simulink model "simple"  (R2016a)
settings: Solver=VariableStepAuto  StartTime=0.0  StopTime=100  FixedStep=0.01  MaxStep=0.01  RelTol=1e-3
undefined symbols (not defined in the file): track_1
libraries: lflib x7
settings Model: Creator=The MathWorks, Inc.  LastModifiedBy=bures
settings SolverCC: ZeroCrossAlgorithm=Adaptive
settings DataIOCC: LimitDataPoints=on
settings DebuggingCC: AllowSymbolicDim=off
settings ModelReferenceCC: PropagateSignalLabelsOutOfModel=off
settings GRTTargetCC: GeneratePreprocessorConditionals=Use local settings

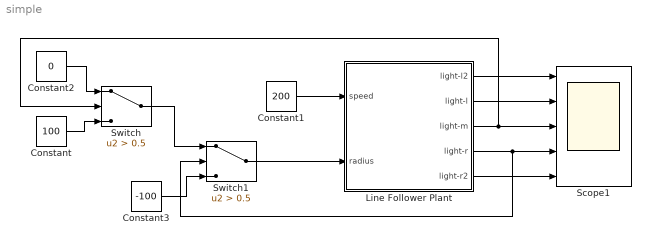
== system simple ==
  Constant : Constant  Value=100
  Constant1 : Constant  Value=200
  Constant2 : Constant  Value=0
  Constant3 : Constant  Value=-100
  Line Follower Plant : Subsystem  mask{initX=506, initY=1050, initAngle=3/2*pi, trackCData=track_1, trackSamplesPerM=1000}
      mask prompts: initX "X (in mm)"; initY "Y (in mm)"; initAngle "Angle (in rad)"; trackCData "Track map"; trackSamplesPerM "Track map samples/m"
  Scope1 : Scope  NumInputPorts=5
  Switch : Switch  Criteria=u2 > Threshold  Threshold=0.5
  Switch1 : Switch  Criteria=u2 > Threshold  Threshold=0.5
  wires:
  Line Follower Plant/1(light-l2) -> Scope1/1
  Line Follower Plant/2(light-l) -> Scope1/2
  Line Follower Plant/5(light-r2) -> Scope1/5
  Line Follower Plant/3(light-m) -> Switch/2, Scope1/3
  Line Follower Plant/4(light-r) -> Switch1/2, Scope1/4
  Switch/1 -> Switch1/1
  Constant1/1 -> Line Follower Plant/1(speed)
  Constant/1 -> Switch/3
  Constant2/1 -> Switch/1
  Constant3/1 -> Switch1/3
  Switch1/1 -> Line Follower Plant/2(radius)

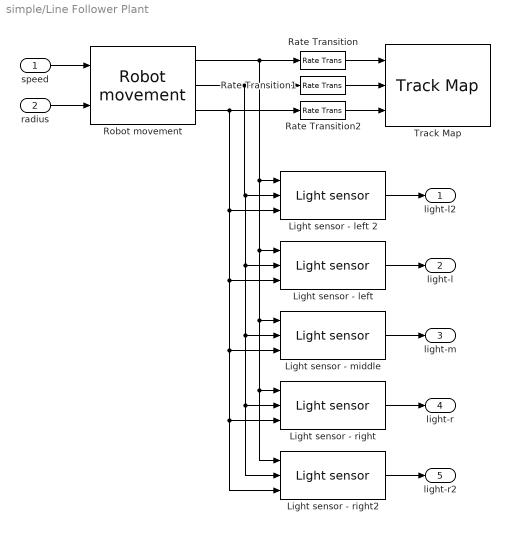
== system simple/Line Follower Plant ==
  speed : Inport
  radius : Inport  Port=2
  Light sensor - left : lflib/Light sensor  trackCData=trackCData  trackSamplesPerM=trackSamplesPerM  sensorPos=[150 30]
  Light sensor - left 2 : lflib/Light sensor  trackCData=trackCData  trackSamplesPerM=trackSamplesPerM  sensorPos=[150 70]
  Light sensor - middle : lflib/Light sensor  trackCData=trackCData  trackSamplesPerM=trackSamplesPerM  sensorPos=[150 0]
  Light sensor - right : lflib/Light sensor  trackCData=trackCData  trackSamplesPerM=trackSamplesPerM  sensorPos=[150 -30]
  Light sensor - right2 : lflib/Light sensor  trackCData=trackCData  trackSamplesPerM=trackSamplesPerM  sensorPos=[150 -70]
  Rate Transition : RateTransition
  Rate Transition1 : RateTransition
  Rate Transition2 : RateTransition
  Robot movement : lflib/Robot movement  initX=initX  initY=initY  initAngle=initAngle
  Track Map : lflib/Track Map  trackCData=trackCData  trackSamplesPerM=trackSamplesPerM
  light-l2 : Outport
  light-l : Outport  Port=2
  light-m : Outport  Port=3
  light-r : Outport  Port=4
  light-r2 : Outport  Port=5
  wires:
  Light sensor - right2/1 -> light-r2/1
  Light sensor - left/1 -> light-l/1
  Light sensor - middle/1 -> light-m/1
  Light sensor - left 2/1 -> light-l2/1
  Light sensor - right/1 -> light-r/1
  Robot movement/1 -> Light sensor - right2/1, Light sensor - right/1, Light sensor - middle/1, Light sensor - left/1, Light sensor - left 2/1, Rate Transition/1
  Robot movement/2 -> Light sensor - right2/2, Light sensor - right/2, Light sensor - middle/2, Light sensor - left/2, Light sensor - left 2/2, Rate Transition1/1
  radius/1 -> Robot movement/2
  speed/1 -> Robot movement/1
  Robot movement/3 -> Light sensor - left/3, Light sensor - middle/3, Light sensor - right/3, Light sensor - right2/3, Light sensor - left 2/3, Rate Transition2/1
  Rate Transition/1 -> Track Map/1
  Rate Transition1/1 -> Track Map/2
  Rate Transition2/1 -> Track Map/3
